simulink model "TPM_Model"  (R2018a)
settings: Solver=ode3  StartTime=0  StopTime=fin  FixedStep=st  MaxStep=0.5  RelTol=1e-3  EnableMultiTasking=on
values from neighbouring files (symbols this model uses):
  A = par(9)    [SPM_Script.m]    (also in TPM_Script.m)
  cs_init_n = x_init * cs_max_n    [SPM_Script.m]    (also in TPM_Script.m = (SOC_p20 * (x100_percent_n - x0_percent_n) + x0_percent_n) *)
  cs_init_p = y_init * cs_max_p    [SPM_Script.m]    (also in TPM_Script.m = (SOC_p20 * (y100_percent_p - y0_percent_p) + y0_percent_p) *)
  del_n = 50e-4    (= 0.005)    [SPM_Script.m]    (also in TPM_Script.m)
  del_p = 36.4e-4    (= 0.00364)    [SPM_Script.m]    (also in TPM_Script.m)
  Ds_n = par(3)    [SPM_Script.m]    (also in TPM_Script.m)
  Ds_p = par(4)    [SPM_Script.m]    (also in TPM_Script.m)
  Farad = 96478    [SPM_Script.m]    (also in TPM_Script.m = 96485)
  par = zeros(11, 1)    [TPM_Script.m]
  Rs_n = 1e-4    (= 0.0001)    [SPM_Script.m]    (also in TPM_Script.m)
  Rs_p = 1e-4    (= 0.0001)    [SPM_Script.m]    (also in TPM_Script.m)
libraries: simulink x1
settings Model: Creator=Cra  LastModifiedBy=jingx
settings DataIOCC: SaveFormat=Array  SignalLoggingSaveFormat=ModelDataLogs  SaveOutput=off  SignalLogging=off
settings OptimizationCC: ExpressionDepthLimit=2147483647  InitFltsAndDblsToZero=on  LifeSpan=inf
settings DebuggingCC: SaveWithParameterizedLinksMsg=none  UnderspecifiedInitializationDetection=Classic  MergeDetectMultiDrivingBlocksExec=none  SolverPrmCheckMsg=warning  FcnCallInpInsideContextMsg=warning  StateNameClashWarn=warning  SFUnexpectedBacktrackingDiag=warning  SFNoUnconditionalDefaultTransitionDiag=warning  SFExecutionAtInitializationDiag=none
settings HardwareCC: ProdBitPerPointer=32  ProdBitPerSizeT=32  ProdBitPerPtrDiffT=32  ProdLargestAtomicFloat=None  ProdIntDivRoundTo=Undefined  ProdEndianess=Unspecified  ProdWordSize=32  ProdHWDeviceType=32-bit Generic
settings ModelReferenceCC: PropagateSignalLabelsOutOfModel=off
settings CodeAppCC: StateflowObjectComments=on
settings GRTTargetCC: TargetFcnLib=ansi_tfl_tmw.mat  TargetLangStandard=C89/C90 (ANSI)  CombineOutputUpdateFcns=off  GRTInterface=on
settings ConfigComp: CovMetricSettings=dw  CovSaveCumulativeToWorkspaceVar=on  CovSaveSingleToWorkspaceVar=on  CovExternalEMLEnable=off

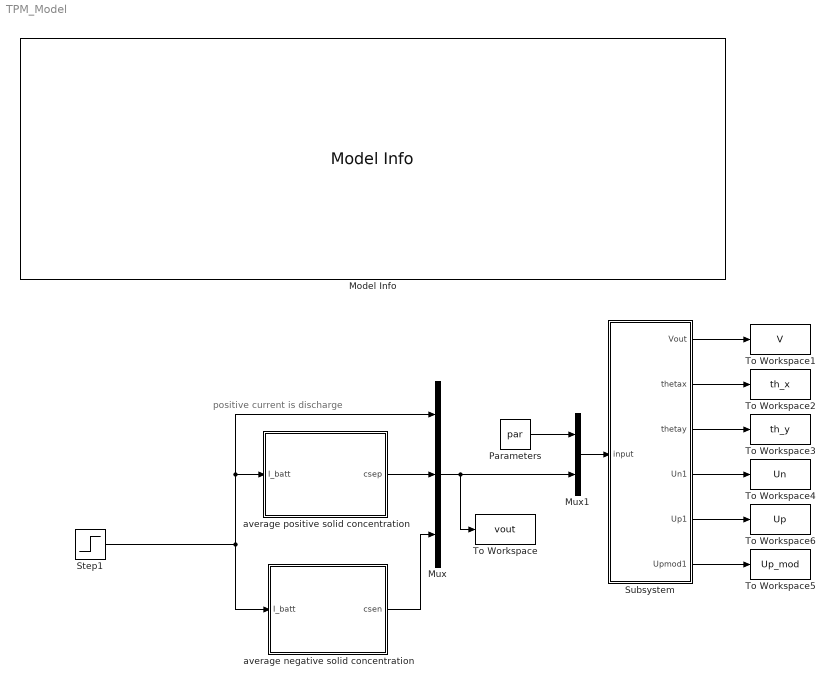
== system TPM_Model ==
  note: positive current is discharge
  Model Info : simulink/Model-Wide Utilities/Model Info  Frame=on  DisplayStringWithTags=|  HorizontalTextAlignment=Left  LeftAlignmentValue=0.02
      | COPYRIGHT  © 2013
      | THE REGENTS OF THE UNIVERSITY OF MICHIGAN
      | ALL RIGHTS RESERVED
      |       
      | PERMISSION IS GRANTED TO USE, COPY, CREATE DERIVATIVE WORKS AND REDISTRIBUTE THIS SOFTWARE AND SUCH DERIVATIVE WORKS FOR NONCOMMERCIAL EDUCATION AND RESEARCH PURPOSES, 
      | SO LONG AS NO FEE IS CHARGED, AND SO LONG AS THE COPYRIGHT NOTICE ABOVE, THIS GRANT OF PERMISSION, AND THE DISCLAIMER BELOW APPEAR IN ALL COPIES MADE; AND SO LONG AS THE NAME 
      | OF THE UNIVERSITY OF MICHIGAN IS NOT USED IN ANY ADVERTISING OR PUBLICITY PERTAINING TO THE USE OR DISTRIBUTION OF THIS SOFTWARE WITHOUT SPECIFIC, WRITTEN PRIOR AUTHORIZATION.
      |     
      | THIS USE OF THIS SOFTWARE REQUIRES SIMULINK, A LICENSED PRODUCT OF THE MATHWORKS, INC.  THE SOFTWARE USER IS SOLELY RESOPNSIBLE FOR OBTAINTING AN APPROPRIATE LICENSE FOR 
      | SIMULINK.  NO LICENSE TO SIMULINK IS GRANTED, INFERRED OR IMPLIED BY THE DISTRIBUTION OF THIS SOFTWARE.
      |     
      | THIS SOFTWARE IS PROVIDED AS IS, WITHOUT REPRESENTATION AS TO ITS FITNESS FOR ANY PURPOSE, AND WITHOUT WARRANTY OF ANY KIND, EITHER EXPRESS OR IMPLIED, INCLUDING WITHOUT 
      | LIMITATION THE IMPLIED WARRANTIES OF MERCHANTABILITY AND FITNESS FOR A PARTICULAR PURPOSE. THE REGENTS OF THE UNIVERSITY OF MICHIGAN SHALL NOT BE LIABLE FOR ANY DAMAGES, 
      | INCLUDING SPECIAL, INDIRECT, INCIDENTAL, OR CONSEQUENTIAL DAMAGES, WITH RESPECT TO ANY CLAIM ARISING OUT OF OR IN CONNECTION WITH THE USE OF THE SOFTWARE, EVEN IF IT HAS 
      | BEEN OR IS HEREAFTER ADVISED OF THE POSSIBILITY OF SUCH DAMAGES.
  Mux : Mux  Inputs=3
  Mux1 : Mux  Inputs=2
  Parameters : Constant  Value=par  VectorParams1D=off
  Step1 : Step  Time=0  After=5  SampleTime=0
  Subsystem : Subsystem
  To Workspace : ToWorkspace  VariableName=vout  SampleTime=-1
  To Workspace1 : ToWorkspace  VariableName=V  SampleTime=-1
  To Workspace2 : ToWorkspace  VariableName=th_x  SampleTime=-1
  To Workspace3 : ToWorkspace  VariableName=th_y  SampleTime=-1
  To Workspace4 : ToWorkspace  VariableName=Un  SampleTime=-1
  To Workspace5 : ToWorkspace  VariableName=Up_mod  SampleTime=-1
  To Workspace6 : ToWorkspace  VariableName=Up  SampleTime=-1
  "average negative solid concentration  " : Subsystem
  average positive solid concentration : Subsystem
  wires:
  average positive solid concentration/1(csep) -> Mux/2
  Mux/1 -> Mux1/2, To Workspace/1
  "average negative solid concentration  "/1(csen) -> Mux/3
  Step1/1 -> Mux/1, average positive solid concentration/1(I_batt), "average negative solid concentration  "/1(I_batt)
  Parameters/1 -> Mux1/1
  Mux1/1 -> Subsystem/1(input)
  Subsystem/1(Vout) -> To Workspace1/1
  Subsystem/2(thetax) -> To Workspace2/1
  Subsystem/3(thetay) -> To Workspace3/1
  Subsystem/4(Un1) -> To Workspace4/1
  Subsystem/5(Up1) -> To Workspace6/1
  Subsystem/6(Upmod1) -> To Workspace5/1

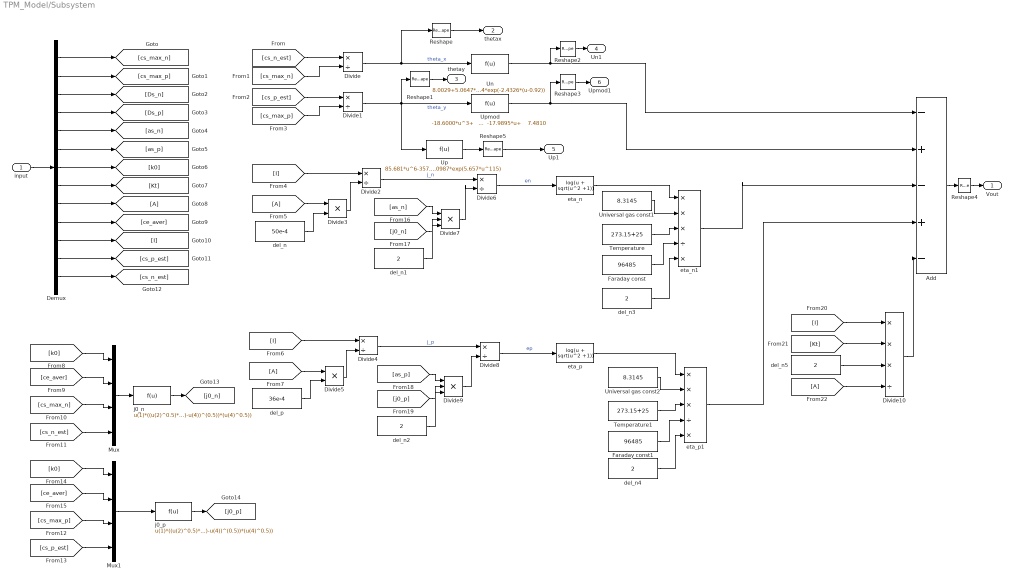
== system TPM_Model/Subsystem ==
  input : Inport
  Add : Sum  Inputs=-+-+-  OutDataTypeStr=double
  Demux : Demux  Outputs=13
  Divide{,1..2,4,6,8} (6 alike) : Product  Inputs=*/
  Divide10 : Product  Inputs=***/
  Divide3 : Product  Inputs=**
  Divide5 : Product  Inputs=**
  Divide7 : Product  Inputs=***
  Divide9 : Product  Inputs=***
  Faraday const : Constant  Value=96485
  Faraday const1 : Constant  Value=96485
  Mux : Mux
  Mux1 : Mux
  Reshape{,1..5} (6 alike) : Reshape
  Temperature : Constant  Value=273.15+25
  Temperature1 : Constant  Value=273.15+25
  Un : Fcn  Expr=8.0029+5.0647*u-12.578*u^0.5-8.6322e-4*u^(-1)+2.1765e-5*u^(3/2)-0.46016*exp(15.0*(0.06-u))-0.55364*exp(-2.4326*(u-0.92))
  Universal gas const1 : Constant  Value=8.3145  VectorParams1D=off
  Universal gas const2 : Constant  Value=8.3145
  Up : Fcn  Expr=85.681*u^6-357.70*u^5+613.89*u^4-555.65*u^3+281.06*u^2-76.648*u+13.1983 -0.30987*exp(5.657*u^115)
  Upmod : Fcn  Expr="-18.6000*u^3+   31.1854*u^2  -17.9895*u+    7.4810"
  del_n : Constant  Value=50e-4
  del_n{1..5} (5 alike) : Constant  Value=2
  del_p : Constant  Value=36e-4
  eta_n : Fcn  Expr=log(u + sqrt(u^2 +1))
  eta_n1 : Product  Inputs=***/*
  eta_p : Fcn  Expr=log(u + sqrt(u^2 +1))
  eta_p1 : Product  Inputs=***/*
  j0_n : Fcn  Expr=u(1)*((u(2)^0.5)*((u(3)-u(4))^(0.5))*(u(4)^0.5))
  j0_p : Fcn  Expr=u(1)*((u(2)^0.5)*((u(3)-u(4))^(0.5))*(u(4)^0.5))
  Vout : Outport  VectorParamsAs1DForOutWhenUnconnected=on
  thetax : Outport  Port=2  VectorParamsAs1DForOutWhenUnconnected=on
  thetay : Outport  Port=3  VectorParamsAs1DForOutWhenUnconnected=on
  Un1 : Outport  Port=4  VectorParamsAs1DForOutWhenUnconnected=on
  Up1 : Outport  Port=5  VectorParamsAs1DForOutWhenUnconnected=on
  Upmod1 : Outport  Port=6  VectorParamsAs1DForOutWhenUnconnected=on
  wires:
  input/1 -> Demux/1
  Demux/1 -> [cs_max_n]
  Demux/2 -> [cs_max_p]
  Demux/3 -> [Ds_n]
  Demux/4 -> [Ds_p]
  Demux/5 -> [as_n]
  Demux/6 -> [as_p]
  Demux/7 -> [k0]
  Demux/8 -> [Kt]
  Demux/9 -> [A]
  Demux/10 -> [ce_aver]
  Demux/11 -> [I]
  Demux/12 -> [cs_p_est]
  Demux/13 -> [cs_n_est]
  [cs_n_est] -> Divide/1
  [cs_max_n] -> Divide/2
  Divide/1 -> Un/1, Reshape/1  "theta_x"
  [cs_p_est] -> Divide1/1
  [cs_max_p] -> Divide1/2
  Divide1/1 -> Upmod/1, Up/1, Reshape1/1  "theta_y"
  [I] -> Divide2/1
  [A] -> Divide3/1
  del_n/1 -> Divide3/2
  Divide3/1 -> Divide2/2
  Divide2/1 -> Divide6/1  "j_n"
  [I] -> Divide4/1
  [A] -> Divide5/1
  del_p/1 -> Divide5/2
  Divide5/1 -> Divide4/2
  Divide4/1 -> Divide8/1  "j_p"
  [k0] -> Mux/1
  [ce_aver] -> Mux/2
  [cs_max_n] -> Mux/3
  [cs_n_est] -> Mux/4
  Mux/1 -> j0_n/1
  [k0] -> Mux1/1
  [ce_aver] -> Mux1/2
  [cs_max_p] -> Mux1/3
  [cs_p_est] -> Mux1/4
  Mux1/1 -> j0_p/1
  [as_n] -> Divide7/1
  [j0_n] -> Divide7/2
  Divide7/1 -> Divide6/2
  j0_n/1 -> [j0_n]
  j0_p/1 -> [j0_p]
  del_n1/1 -> Divide7/3
  [as_p] -> Divide9/1
  [j0_p] -> Divide9/2
  Divide9/1 -> Divide8/2
  del_n2/1 -> Divide9/3
  Divide6/1 -> eta_n/1  "en"
  Divide8/1 -> eta_p/1  "ep"
  Universal gas const1/1 -> eta_n1/2
  Temperature/1 -> eta_n1/3
  Faraday const/1 -> eta_n1/4
  Universal gas const2/1 -> eta_p1/2
  Temperature1/1 -> eta_p1/3
  Faraday const1/1 -> eta_p1/4
  del_n4/1 -> eta_p1/5
  eta_p/1 -> eta_p1/1
  del_n3/1 -> eta_n1/5
  eta_n/1 -> eta_n1/1
  Un/1 -> Add/1, Reshape2/1
  Upmod/1 -> Add/2, Reshape3/1
  eta_n1/1 -> Add/3
  eta_p1/1 -> Add/4
  [I] -> Divide10/1
  [Kt] -> Divide10/2
  del_n5/1 -> Divide10/3
  [A] -> Divide10/4
  Divide10/1 -> Add/5
  Add/1 -> Reshape4/1
  Up/1 -> Reshape5/1
  Reshape/1 -> thetax/1
  Reshape1/1 -> thetay/1
  Reshape2/1 -> Un1/1
  Reshape3/1 -> Upmod1/1
  Reshape4/1 -> Vout/1
  Reshape5/1 -> Up1/1

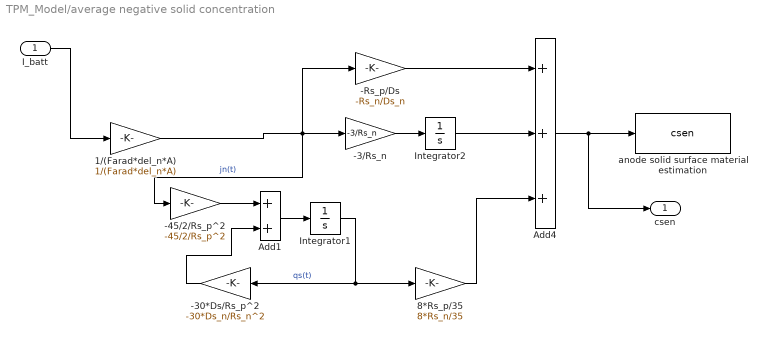
== system TPM_Model/average negative solid concentration   ==
  I_batt : Inport
  -3/Rs_n : Gain  Gain=-3/Rs_n
  -30*Ds/Rs_p^2 : Gain  Gain=-30*Ds_n/Rs_n^2
  -45/2/Rs_p^2 : Gain  Gain=-45/2/Rs_p^2
  -Rs_p/Ds : Gain  Gain=-Rs_n/Ds_n
  1/(Farad*del_n*A) : Gain  Gain=1/(Farad*del_n*A)
  8*Rs_p/35 : Gain  Gain=8*Rs_n/35
  Add1 : Sum
  Add4 : Sum  Inputs=+++
  Integrator1 : Integrator  InitialCondition=cs_init_n
  Integrator2 : Integrator  InitialCondition=cs_init_n
  anode solid surface material estimation : ToWorkspace  VariableName=csen  SampleTime=-1
  csen : Outport  VectorParamsAs1DForOutWhenUnconnected=on
  wires:
  1/(Farad*del_n*A)/1 -> -3/Rs_n/1, -Rs_p/Ds/1, -45/2/Rs_p^2/1  "jn(t)"
  -Rs_p/Ds/1 -> Add4/1
  Add4/1 -> anode solid surface material estimation/1, csen/1
  I_batt/1 -> 1/(Farad*del_n*A)/1
  -45/2/Rs_p^2/1 -> Add1/1
  Add1/1 -> Integrator1/1
  Integrator1/1 -> 8*Rs_p/35/1, -30*Ds/Rs_p^2/1  "qs(t)"
  -30*Ds/Rs_p^2/1 -> Add1/2
  8*Rs_p/35/1 -> Add4/3
  Integrator2/1 -> Add4/2
  -3/Rs_n/1 -> Integrator2/1

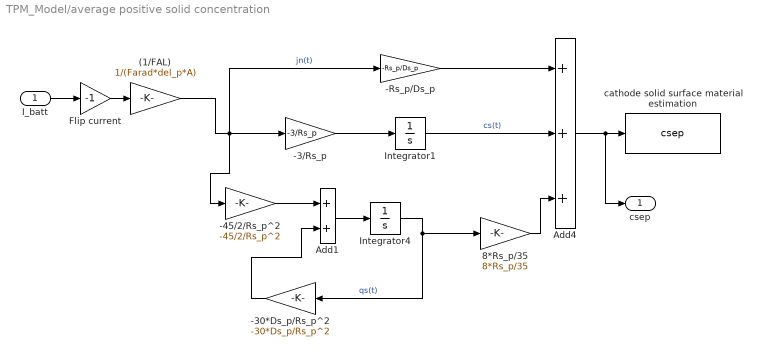
== system TPM_Model/average positive solid concentration ==
  I_batt : Inport
  (1/FAL) : Gain  Gain=1/(Farad*del_p*A)
  "-3/Rs_p " : Gain  Gain=-3/Rs_p
  -30*Ds_p/Rs_p^2 : Gain  Gain=-30*Ds_p/Rs_p^2
  -45/2/Rs_p^2 : Gain  Gain=-45/2/Rs_p^2
  -Rs_p/Ds_p : Gain  Gain=-Rs_p/Ds_p
  8*Rs_p/35 : Gain  Gain=8*Rs_p/35
  Add1 : Sum
  Add4 : Sum  Inputs=+++
  Flip current : Gain  Gain=-1
  Integrator1 : Integrator  InitialCondition=cs_init_p  LimitOutput=on
  Integrator4 : Integrator  InitialCondition=cs_init_p  LimitOutput=on
  cathode solid surface material estimation : ToWorkspace  VariableName=csep  SampleTime=-1
  csep : Outport  VectorParamsAs1DForOutWhenUnconnected=on
  wires:
  Add4/1 -> cathode solid surface material estimation/1, csep/1
  Flip current/1 -> (1/FAL)/1
  I_batt/1 -> Flip current/1
  (1/FAL)/1 -> -45/2/Rs_p^2/1, "-3/Rs_p "/1, -Rs_p/Ds_p/1  "jn(t)"
  Integrator1/1 -> Add4/2  "cs(t)"
  -Rs_p/Ds_p/1 -> Add4/1
  -45/2/Rs_p^2/1 -> Add1/1
  Add1/1 -> Integrator4/1
  -30*Ds_p/Rs_p^2/1 -> Add1/2
  Integrator4/1 -> -30*Ds_p/Rs_p^2/1, 8*Rs_p/35/1  "qs(t)"
  8*Rs_p/35/1 -> Add4/3
  "-3/Rs_p "/1 -> Integrator1/1
